simulink library "halout"  (R2021b)
settings: Solver=VariableStepAuto  StartTime=0.0  StopTime=10.0  RelTol=1e-3
undefined symbols (not defined in the file): C_TASK_5MS_S, FALSE, KHAL_CAN1FD1APS3E2E_flg, KHAL_CAN1FD1APS3TxReq_flg, KHAL_CAN1FD1VCU2E2E_flg, KHAL_CAN1FD1VCU2TxReq_flg, KHAL_CAN1FD1VCU3E2E_flg, KHAL_CAN1FD1VCU3TxReq_flg, KHAL_CAN1TxReq_flg, KHAL_CAN1VMCFCM1E2E_flg, KHAL_CAN1VMCFCM1TxReq_flg, KHAL_CAN2TxReq_flg, KHAL_CAN3FD3VCU1toNIDECTxReq_flg, KHAL_CAN3FD3VCU1TxReq_flg, KHAL_CAN3FD3VCU2E2E_flg, KHAL_CAN3FD3VCU2toNIDECE2E_flg, KHAL_CAN3FD3VCU2toNIDECTxReq_flg, KHAL_CAN3FD3VCU2TxReq_flg, KHAL_CAN3TxReq_flg, KHAL_CAN4FD4CE1000E2E_flg, KHAL_CAN4FD4CE1000TxReq_flg, KHAL_CAN4TxReq_flg, KHAL_CAN5TxReq_flg, KHAL_CAN6FD6APS3E2E_flg, KHAL_CAN6FD6APS3TxReq_flg, KHAL_CAN6FD6VCU2E2E_flg, KHAL_CAN6FD6VCU2TxReq_flg, KHAL_CAN6TxReq_flg, ONE_INT, TRUE, ZERO_INT
libraries: FVT_lib x551, simulink x244
(part 24 of 26)

== system halout/HAL_OUT/CAN5/FD5_Debug2_0x4F7/FDCDKCRemoRightPSDCmd ==
  FDCDKCRemoRightPSDCmd : Inport
  Data Type Conversion : DataTypeConversion  OutDataTypeStr=uint8  RndMeth=Round
  CAN5_FDC_DKC_RemoRightPSD_Cmd : Outport
  wires:
  Data Type Conversion/1 -> CAN5_FDC_DKC_RemoRightPSD_Cmd/1
  FDCDKCRemoRightPSDCmd/1 -> Data Type Conversion/1

== system halout/HAL_OUT/CAN5/FD5_Debug2_0x4F7/FDCDKCSPTGDetCmd ==
  FDCDKCSPTGDetCmd : Inport
  Data Type Conversion : DataTypeConversion  OutDataTypeStr=uint8  RndMeth=Round
  CAN5_FDC_DKC_SPTGDet_Cmd : Outport
  wires:
  Data Type Conversion/1 -> CAN5_FDC_DKC_SPTGDet_Cmd/1
  FDCDKCSPTGDetCmd/1 -> Data Type Conversion/1

== system halout/HAL_OUT/CAN5/FD5_Debug2_0x4F7/FDCDKCSPTGOpenCmd ==
  FDCDKCSPTGOpenCmd : Inport
  Data Type Conversion : DataTypeConversion  OutDataTypeStr=uint8  RndMeth=Round
  CAN5_FDC_DKC_SPTGOpen_Cmd : Outport
  wires:
  Data Type Conversion/1 -> CAN5_FDC_DKC_SPTGOpen_Cmd/1
  FDCDKCSPTGOpenCmd/1 -> Data Type Conversion/1

== system halout/HAL_OUT/CAN5/FD5_Debug2_0x4F7/FDCDKCShippingModeSta ==
  FDCDKCShippingModeSta : Inport
  Data Type Conversion : DataTypeConversion  OutDataTypeStr=uint8  RndMeth=Round
  CAN5_FDC_DKC_ShippingMode_Sta : Outport
  wires:
  Data Type Conversion/1 -> CAN5_FDC_DKC_ShippingMode_Sta/1
  FDCDKCShippingModeSta/1 -> Data Type Conversion/1

== system halout/HAL_OUT/CAN5/FD5_Debug2_0x4F7/FDCDKCUIDBatVoltSta ==
  FDCDKCUIDBatVoltSta : Inport
  Data Type Conversion : DataTypeConversion  OutDataTypeStr=uint16  RndMeth=Round
  convert_out : FVT_lib/hal/convert_out  gain=10  offset=0
  CAN5_FDC_DKC_UIDBatVolt_Sta : Outport
  wires:
  Data Type Conversion/1 -> CAN5_FDC_DKC_UIDBatVolt_Sta/1
  convert_out/1 -> Data Type Conversion/1
  FDCDKCUIDBatVoltSta/1 -> convert_out/1

== system halout/HAL_OUT/CAN5/FD5_Debug2_0x4F7/FDCDKCUIDLowPowerSta ==
  FDCDKCUIDLowPowerSta : Inport
  Data Type Conversion : DataTypeConversion  OutDataTypeStr=uint8  RndMeth=Round
  CAN5_FDC_DKC_UIDLowPower_Sta : Outport
  wires:
  Data Type Conversion/1 -> CAN5_FDC_DKC_UIDLowPower_Sta/1
  FDCDKCUIDLowPowerSta/1 -> Data Type Conversion/1

== system halout/HAL_OUT/CAN5/FD5_Debug2_0x4F7/FDCDKCUWB1DistanceSta ==
  FDCDKCUWB1DistanceSta : Inport
  Data Type Conversion : DataTypeConversion  OutDataTypeStr=uint8  RndMeth=Round
  convert_out : FVT_lib/hal/convert_out  gain=10  offset=0
  CAN5_FDC_DKC_UWB1_Distance_Sta : Outport
  wires:
  Data Type Conversion/1 -> CAN5_FDC_DKC_UWB1_Distance_Sta/1
  convert_out/1 -> Data Type Conversion/1
  FDCDKCUWB1DistanceSta/1 -> convert_out/1

== system halout/HAL_OUT/CAN5/FD5_Debug2_0x4F7/FDCDKCUWB1FPPSta ==
  FDCDKCUWB1FPPSta : Inport
  Data Type Conversion : DataTypeConversion  OutDataTypeStr=uint8  RndMeth=Round
  convert_out : FVT_lib/hal/convert_out  gain=1  offset=-127
  CAN5_FDC_DKC_UWB1_FPP_Sta : Outport
  wires:
  Data Type Conversion/1 -> CAN5_FDC_DKC_UWB1_FPP_Sta/1
  convert_out/1 -> Data Type Conversion/1
  FDCDKCUWB1FPPSta/1 -> convert_out/1

== system halout/HAL_OUT/CAN5/FD5_Debug2_0x4F7/FDCDKCUWB1InvalidSta ==
  FDCDKCUWB1InvalidSta : Inport
  Data Type Conversion : DataTypeConversion  OutDataTypeStr=uint8  RndMeth=Round
  CAN5_FDC_DKC_UWB1_Invalid_Sta : Outport
  wires:
  Data Type Conversion/1 -> CAN5_FDC_DKC_UWB1_Invalid_Sta/1
  FDCDKCUWB1InvalidSta/1 -> Data Type Conversion/1

== system halout/HAL_OUT/CAN5/FD5_Debug2_0x4F7/FDCDKCUWB2DistanceSta ==
  FDCDKCUWB2DistanceSta : Inport
  Data Type Conversion : DataTypeConversion  OutDataTypeStr=uint8  RndMeth=Round
  convert_out : FVT_lib/hal/convert_out  gain=10  offset=0
  CAN5_FDC_DKC_UWB2_Distance_Sta : Outport
  wires:
  Data Type Conversion/1 -> CAN5_FDC_DKC_UWB2_Distance_Sta/1
  convert_out/1 -> Data Type Conversion/1
  FDCDKCUWB2DistanceSta/1 -> convert_out/1

== system halout/HAL_OUT/CAN5/FD5_Debug2_0x4F7/FDCDKCUWB2FPPSta ==
  FDCDKCUWB2FPPSta : Inport
  Data Type Conversion : DataTypeConversion  OutDataTypeStr=uint8  RndMeth=Round
  convert_out : FVT_lib/hal/convert_out  gain=1  offset=-127
  CAN5_FDC_DKC_UWB2_FPP_Sta : Outport
  wires:
  Data Type Conversion/1 -> CAN5_FDC_DKC_UWB2_FPP_Sta/1
  convert_out/1 -> Data Type Conversion/1
  FDCDKCUWB2FPPSta/1 -> convert_out/1

== system halout/HAL_OUT/CAN5/FD5_Debug2_0x4F7/FDCDKCUWB2InvalidSta ==
  FDCDKCUWB2InvalidSta : Inport
  Data Type Conversion : DataTypeConversion  OutDataTypeStr=uint8  RndMeth=Round
  CAN5_FDC_DKC_UWB2_Invalid_Sta : Outport
  wires:
  Data Type Conversion/1 -> CAN5_FDC_DKC_UWB2_Invalid_Sta/1
  FDCDKCUWB2InvalidSta/1 -> Data Type Conversion/1

== system halout/HAL_OUT/CAN5/FD5_Debug2_0x4F7/FDCDKCUWB3DistanceSta ==
  FDCDKCUWB3DistanceSta : Inport
  Data Type Conversion : DataTypeConversion  OutDataTypeStr=uint8  RndMeth=Round
  convert_out : FVT_lib/hal/convert_out  gain=10  offset=0
  CAN5_FDC_DKC_UWB3_Distance_Sta : Outport
  wires:
  Data Type Conversion/1 -> CAN5_FDC_DKC_UWB3_Distance_Sta/1
  convert_out/1 -> Data Type Conversion/1
  FDCDKCUWB3DistanceSta/1 -> convert_out/1

== system halout/HAL_OUT/CAN5/FD5_Debug2_0x4F7/FDCDKCUWB3FPPSta ==
  FDCDKCUWB3FPPSta : Inport
  Data Type Conversion : DataTypeConversion  OutDataTypeStr=uint8  RndMeth=Round
  convert_out : FVT_lib/hal/convert_out  gain=1  offset=-127
  CAN5_FDC_DKC_UWB3_FPP_Sta : Outport
  wires:
  Data Type Conversion/1 -> CAN5_FDC_DKC_UWB3_FPP_Sta/1
  convert_out/1 -> Data Type Conversion/1
  FDCDKCUWB3FPPSta/1 -> convert_out/1

== system halout/HAL_OUT/CAN5/FD5_Debug2_0x4F7/FDCDKCUWB3InvalidSta ==
  FDCDKCUWB3InvalidSta : Inport
  Data Type Conversion : DataTypeConversion  OutDataTypeStr=uint8  RndMeth=Round
  CAN5_FDC_DKC_UWB3_Invalid_Sta : Outport
  wires:
  Data Type Conversion/1 -> CAN5_FDC_DKC_UWB3_Invalid_Sta/1
  FDCDKCUWB3InvalidSta/1 -> Data Type Conversion/1

== system halout/HAL_OUT/CAN5/FD5_Debug2_0x4F7/FDCDKCUWB4DistanceSta ==
  FDCDKCUWB4DistanceSta : Inport
  Data Type Conversion : DataTypeConversion  OutDataTypeStr=uint8  RndMeth=Round
  convert_out : FVT_lib/hal/convert_out  gain=10  offset=0
  CAN5_FDC_DKC_UWB4_Distance_Sta : Outport
  wires:
  Data Type Conversion/1 -> CAN5_FDC_DKC_UWB4_Distance_Sta/1
  convert_out/1 -> Data Type Conversion/1
  FDCDKCUWB4DistanceSta/1 -> convert_out/1

== system halout/HAL_OUT/CAN5/FD5_Debug2_0x4F7/FDCDKCUWB4FPPSta ==
  FDCDKCUWB4FPPSta : Inport
  Data Type Conversion : DataTypeConversion  OutDataTypeStr=uint8  RndMeth=Round
  convert_out : FVT_lib/hal/convert_out  gain=1  offset=-127
  CAN5_FDC_DKC_UWB4_FPP_Sta : Outport
  wires:
  Data Type Conversion/1 -> CAN5_FDC_DKC_UWB4_FPP_Sta/1
  convert_out/1 -> Data Type Conversion/1
  FDCDKCUWB4FPPSta/1 -> convert_out/1

== system halout/HAL_OUT/CAN5/FD5_Debug2_0x4F7/FDCDKCUWB4InvalidSta ==
  FDCDKCUWB4InvalidSta : Inport
  Data Type Conversion : DataTypeConversion  OutDataTypeStr=uint8  RndMeth=Round
  CAN5_FDC_DKC_UWB4_Invalid_Sta : Outport
  wires:
  Data Type Conversion/1 -> CAN5_FDC_DKC_UWB4_Invalid_Sta/1
  FDCDKCUWB4InvalidSta/1 -> Data Type Conversion/1

== system halout/HAL_OUT/CAN5/FD5_Debug2_0x4F7/FDCDKCUWB5DistanceSta ==
  FDCDKCUWB5DistanceSta : Inport
  Data Type Conversion : DataTypeConversion  OutDataTypeStr=uint8  RndMeth=Round
  convert_out : FVT_lib/hal/convert_out  gain=10  offset=0
  CAN5_FDC_DKC_UWB5_Distance_Sta : Outport
  wires:
  Data Type Conversion/1 -> CAN5_FDC_DKC_UWB5_Distance_Sta/1
  convert_out/1 -> Data Type Conversion/1
  FDCDKCUWB5DistanceSta/1 -> convert_out/1

== system halout/HAL_OUT/CAN5/FD5_Debug2_0x4F7/FDCDKCUWB5FPPSta ==
  FDCDKCUWB5FPPSta : Inport
  Data Type Conversion : DataTypeConversion  OutDataTypeStr=uint8  RndMeth=Round
  convert_out : FVT_lib/hal/convert_out  gain=1  offset=-127
  CAN5_FDC_DKC_UWB5_FPP_Sta : Outport
  wires:
  Data Type Conversion/1 -> CAN5_FDC_DKC_UWB5_FPP_Sta/1
  convert_out/1 -> Data Type Conversion/1
  FDCDKCUWB5FPPSta/1 -> convert_out/1

== system halout/HAL_OUT/CAN5/FD5_Debug2_0x4F7/FDCDKCUWB5InvalidSta ==
  FDCDKCUWB5InvalidSta : Inport
  Data Type Conversion : DataTypeConversion  OutDataTypeStr=uint8  RndMeth=Round
  CAN5_FDC_DKC_UWB5_Invalid_Sta : Outport
  wires:
  Data Type Conversion/1 -> CAN5_FDC_DKC_UWB5_Invalid_Sta/1
  FDCDKCUWB5InvalidSta/1 -> Data Type Conversion/1

== system halout/HAL_OUT/CAN5/FD5_Debug2_0x4F7/FDCDKCUWBDetAreaSta ==
  FDCDKCUWBDetAreaSta : Inport
  Data Type Conversion : DataTypeConversion  OutDataTypeStr=uint8  RndMeth=Round
  CAN5_FDC_DKC_UWBDetArea_Sta : Outport
  wires:
  Data Type Conversion/1 -> CAN5_FDC_DKC_UWBDetArea_Sta/1
  FDCDKCUWBDetAreaSta/1 -> Data Type Conversion/1

== system halout/HAL_OUT/CAN5/FD5_Debug2_0x4F7/FDCDKCUWBDetPTGAreaSta ==
  FDCDKCUWBDetPTGAreaSta : Inport
  Data Type Conversion : DataTypeConversion  OutDataTypeStr=uint8  RndMeth=Round
  CAN5_FDC_DKC_UWBDetPTGArea_Sta : Outport
  wires:
  Data Type Conversion/1 -> CAN5_FDC_DKC_UWBDetPTGArea_Sta/1
  FDCDKCUWBDetPTGAreaSta/1 -> Data Type Conversion/1

== system halout/HAL_OUT/CAN5/FD5_Debug2_0x4F7/FDCDKCUWBOnOffSta ==
  FDCDKCUWBOnOffSta : Inport
  Data Type Conversion : DataTypeConversion  OutDataTypeStr=uint8  RndMeth=Round
  CAN5_FDC_DKC_UWB_OnOff_Sta : Outport
  wires:
  Data Type Conversion/1 -> CAN5_FDC_DKC_UWB_OnOff_Sta/1
  FDCDKCUWBOnOffSta/1 -> Data Type Conversion/1

== system halout/HAL_OUT/CAN5/FD5_Debug3_0x4F3/FDCVMCActReqAccCmd ==
  FDCVMCActReqAccCmd : Inport
  Data Type Conversion : DataTypeConversion  OutDataTypeStr=uint16  RndMeth=Round
  convert_out : FVT_lib/hal/convert_out  gain=0.05  offset=-15
  CAN5_FDC_VMC_ActReqAcc_Cmd : Outport
  wires:
  Data Type Conversion/1 -> CAN5_FDC_VMC_ActReqAcc_Cmd/1
  convert_out/1 -> Data Type Conversion/1
  FDCVMCActReqAccCmd/1 -> convert_out/1

== system halout/HAL_OUT/CAN5/FD5_Debug3_0x4F3/FDCVMCExtraMSACtrlSta ==
  FDCVMCExtraMSACtrlSta : Inport
  Data Type Conversion : DataTypeConversion  OutDataTypeStr=uint8  RndMeth=Round
  CAN5_FDC_VMC_ExtraMSACtrl_Sta : Outport
  wires:
  Data Type Conversion/1 -> CAN5_FDC_VMC_ExtraMSACtrl_Sta/1
  FDCVMCExtraMSACtrlSta/1 -> Data Type Conversion/1

== system halout/HAL_OUT/CAN5/FD5_Debug3_0x4F3/FDCVMCIMUGxCmd ==
  FDCVMCIMUGxCmd : Inport
  Data Type Conversion : DataTypeConversion  OutDataTypeStr=uint8  RndMeth=Round
  convert_out : FVT_lib/hal/convert_out  gain=0.01  offset=-1.27
  CAN5_FDC_VMC_IMUGx_Cmd : Outport
  wires:
  Data Type Conversion/1 -> CAN5_FDC_VMC_IMUGx_Cmd/1
  convert_out/1 -> Data Type Conversion/1
  FDCVMCIMUGxCmd/1 -> convert_out/1

== system halout/HAL_OUT/CAN5/FD5_Debug3_0x4F3/FDCVMCIMUGyCmd ==
  FDCVMCIMUGyCmd : Inport
  Data Type Conversion : DataTypeConversion  OutDataTypeStr=uint8  RndMeth=Round
  convert_out : FVT_lib/hal/convert_out  gain=0.01  offset=-1.27
  CAN5_FDC_VMC_IMUGy_Cmd : Outport
  wires:
  Data Type Conversion/1 -> CAN5_FDC_VMC_IMUGy_Cmd/1
  convert_out/1 -> Data Type Conversion/1
  FDCVMCIMUGyCmd/1 -> convert_out/1

== system halout/HAL_OUT/CAN5/FD5_Debug3_0x4F3/FDCVMCIMUGzCmd ==
  FDCVMCIMUGzCmd : Inport
  Data Type Conversion : DataTypeConversion  OutDataTypeStr=uint8  RndMeth=Round
  convert_out : FVT_lib/hal/convert_out  gain=0.01  offset=-1.27
  CAN5_FDC_VMC_IMUGz_Cmd : Outport
  wires:
  Data Type Conversion/1 -> CAN5_FDC_VMC_IMUGz_Cmd/1
  convert_out/1 -> Data Type Conversion/1
  FDCVMCIMUGzCmd/1 -> convert_out/1

== system halout/HAL_OUT/CAN5/FD5_Debug3_0x4F3/FDCVMCIMUPitchRateCmd ==
  FDCVMCIMUPitchRateCmd : Inport
  Data Type Conversion : DataTypeConversion  OutDataTypeStr=uint16  RndMeth=Round
  convert_out : FVT_lib/hal/convert_out  gain=0.1  offset=-100
  CAN5_FDC_VMC_IMUPitchRate_Cmd : Outport
  wires:
  Data Type Conversion/1 -> CAN5_FDC_VMC_IMUPitchRate_Cmd/1
  convert_out/1 -> Data Type Conversion/1
  FDCVMCIMUPitchRateCmd/1 -> convert_out/1

== system halout/HAL_OUT/CAN5/FD5_Debug3_0x4F3/FDCVMCIMURollRateCmd ==
  FDCVMCIMURollRateCmd : Inport
  Data Type Conversion : DataTypeConversion  OutDataTypeStr=uint16  RndMeth=Round
  convert_out : FVT_lib/hal/convert_out  gain=0.1  offset=-100
  CAN5_FDC_VMC_IMURollRate_Cmd : Outport
  wires:
  Data Type Conversion/1 -> CAN5_FDC_VMC_IMURollRate_Cmd/1
  convert_out/1 -> Data Type Conversion/1
  FDCVMCIMURollRateCmd/1 -> convert_out/1

== system halout/HAL_OUT/CAN5/FD5_Debug3_0x4F3/FDCVMCIMUYawRateCmd ==
  FDCVMCIMUYawRateCmd : Inport
  Data Type Conversion : DataTypeConversion  OutDataTypeStr=uint16  RndMeth=Round
  convert_out : FVT_lib/hal/convert_out  gain=0.1  offset=-100
  CAN5_FDC_VMC_IMUYawRate_Cmd : Outport
  wires:
  Data Type Conversion/1 -> CAN5_FDC_VMC_IMUYawRate_Cmd/1
  convert_out/1 -> Data Type Conversion/1
  FDCVMCIMUYawRateCmd/1 -> convert_out/1

== system halout/HAL_OUT/CAN5/FD5_Debug3_0x4F3/FDCVMCLongAccelCmd ==
  FDCVMCLongAccelCmd : Inport
  Data Type Conversion : DataTypeConversion  OutDataTypeStr=uint8  RndMeth=Round
  convert_out : FVT_lib/hal/convert_out  gain=0.01  offset=-1.27
  CAN5_FDC_VMC_LongAccel_Cmd : Outport
  wires:
  Data Type Conversion/1 -> CAN5_FDC_VMC_LongAccel_Cmd/1
  convert_out/1 -> Data Type Conversion/1
  FDCVMCLongAccelCmd/1 -> convert_out/1

== system halout/HAL_OUT/CAN5/GW5_CE100_0_0x1C5/FDCBCMWinLFOpenedSta ==
  FDCBCMWinLFOpenedSta : Inport
  Data Type Conversion : DataTypeConversion  OutDataTypeStr=uint8  RndMeth=Round
  CAN5_FDC_BCM_WinLFOpened_Sta : Outport
  wires:
  Data Type Conversion/1 -> CAN5_FDC_BCM_WinLFOpened_Sta/1
  FDCBCMWinLFOpenedSta/1 -> Data Type Conversion/1

== system halout/HAL_OUT/CAN5/GW5_CE100_0_0x1C5/FDCBCMWinLROpenedSta ==
  FDCBCMWinLROpenedSta : Inport
  Data Type Conversion : DataTypeConversion  OutDataTypeStr=uint8  RndMeth=Round
  CAN5_FDC_BCM_WinLROpened_Sta : Outport
  wires:
  Data Type Conversion/1 -> CAN5_FDC_BCM_WinLROpened_Sta/1
  FDCBCMWinLROpenedSta/1 -> Data Type Conversion/1

== system halout/HAL_OUT/CAN5/GW5_CE100_0_0x1C5/FDCBCMWinRFOpenedSta ==
  FDCBCMWinRFOpenedSta : Inport
  Data Type Conversion : DataTypeConversion  OutDataTypeStr=uint8  RndMeth=Round
  CAN5_FDC_BCM_WinRFOpened_Sta : Outport
  wires:
  Data Type Conversion/1 -> CAN5_FDC_BCM_WinRFOpened_Sta/1
  FDCBCMWinRFOpenedSta/1 -> Data Type Conversion/1

== system halout/HAL_OUT/CAN5/GW5_CE100_0_0x1C5/FDCBCMWinRROpenedSta ==
  FDCBCMWinRROpenedSta : Inport
  Data Type Conversion : DataTypeConversion  OutDataTypeStr=uint8  RndMeth=Round
  CAN5_FDC_BCM_WinRROpened_Sta : Outport
  wires:
  Data Type Conversion/1 -> CAN5_FDC_BCM_WinRROpened_Sta/1
  FDCBCMWinRROpenedSta/1 -> Data Type Conversion/1

== system halout/HAL_OUT/CAN6/FD6_APS3_0x238/APS3LifeCount ==
  APS3LifeCount : Inport
  Data Type Conversion : DataTypeConversion  OutDataTypeStr=uint8  RndMeth=Round
  CAN6_APS3_LifeCount : Outport
  wires:
  Data Type Conversion/1 -> CAN6_APS3_LifeCount/1
  APS3LifeCount/1 -> Data Type Conversion/1

== system halout/HAL_OUT/CAN6/FD6_APS3_0x238/APS3checksum ==
  APS3checksum : Inport
  Data Type Conversion : DataTypeConversion  OutDataTypeStr=uint8  RndMeth=Round
  CAN6_APS3_checksum : Outport
  wires:
  Data Type Conversion/1 -> CAN6_APS3_checksum/1
  APS3checksum/1 -> Data Type Conversion/1

== system halout/HAL_OUT/CAN6/FD6_APS3_0x238/APSDecReq ==
  APSDecReq : Inport
  Data Type Conversion : DataTypeConversion  OutDataTypeStr=uint8  RndMeth=Round
  convert_out : FVT_lib/hal/convert_out  gain=0.1  offset=0
  CAN6_APS_DecReq : Outport
  wires:
  Data Type Conversion/1 -> CAN6_APS_DecReq/1
  convert_out/1 -> Data Type Conversion/1
  APSDecReq/1 -> convert_out/1

== system halout/HAL_OUT/CAN6/FD6_APS3_0x238/APSDecReqA ==
  APSDecReqA : Inport
  Data Type Conversion : DataTypeConversion  OutDataTypeStr=uint8  RndMeth=Round
  CAN6_APS_DecReq_A : Outport
  wires:
  Data Type Conversion/1 -> CAN6_APS_DecReq_A/1
  APSDecReqA/1 -> Data Type Conversion/1

== system halout/HAL_OUT/CAN6/FD6_APS3_0x238/APSOpenPTG ==
  APSOpenPTG : Inport
  Data Type Conversion : DataTypeConversion  OutDataTypeStr=uint8  RndMeth=Round
  CAN6_APSOpenPTG : Outport
  wires:
  Data Type Conversion/1 -> CAN6_APSOpenPTG/1
  APSOpenPTG/1 -> Data Type Conversion/1

== system halout/HAL_OUT/CAN6/FD6_APS3_0x238/APSReq ==
  APSReq : Inport
  Data Type Conversion : DataTypeConversion  OutDataTypeStr=uint8  RndMeth=Round
  CAN6_APS_Req : Outport
  wires:
  Data Type Conversion/1 -> CAN6_APS_Req/1
  APSReq/1 -> Data Type Conversion/1

== system halout/HAL_OUT/CAN6/FD6_APS3_0x238/APSStaSystem ==
  APSStaSystem : Inport
  Data Type Conversion : DataTypeConversion  OutDataTypeStr=uint8  RndMeth=Round
  CAN6_APS_Sta_System : Outport
  wires:
  Data Type Conversion/1 -> CAN6_APS_Sta_System/1
  APSStaSystem/1 -> Data Type Conversion/1

== system halout/HAL_OUT/CAN6/FD6_APS3_0x238/Byte_0 ==
  APS3_checksum : Inport
  BitwiseOR : simulink/Logic and Bit Operations/Bitwise Operator  logicop=OR  UseBitMask=off  BitMask=bin2dec('11011001')  BitMaskRealWorld=Stored Integer
  SignalPack : FVT_lib/hal/SignalPack  RightShiftCnt=0  BitMask=2^8-1  LeftShiftCnt=0
  UnitConverter : DataTypeConversion  OutDataTypeStr=uint8  RndMeth=Round
  UnitConverter1 : DataTypeConversion  OutDataTypeStr=uint8  RndMeth=Round
  Byte_0 : Outport
  wires:
  BitwiseOR/1 -> Byte_0/1
  UnitConverter/1 -> BitwiseOR/1
  SignalPack/1 -> UnitConverter/1
  UnitConverter1/1 -> SignalPack/1
  APS3_checksum/1 -> UnitConverter1/1

== system halout/HAL_OUT/CAN6/FD6_APS3_0x238/Byte_1 ==
  APS3_LifeCount : Inport
  BitwiseOR : simulink/Logic and Bit Operations/Bitwise Operator  logicop=OR  UseBitMask=off  BitMask=bin2dec('11011001')  BitMaskRealWorld=Stored Integer
  SignalPack : FVT_lib/hal/SignalPack  RightShiftCnt=0  BitMask=2^4-1  LeftShiftCnt=0
  UnitConverter : DataTypeConversion  OutDataTypeStr=uint8  RndMeth=Round
  UnitConverter1 : DataTypeConversion  OutDataTypeStr=uint8  RndMeth=Round
  Byte_1 : Outport
  wires:
  BitwiseOR/1 -> Byte_1/1
  UnitConverter/1 -> BitwiseOR/1
  SignalPack/1 -> UnitConverter/1
  UnitConverter1/1 -> SignalPack/1
  APS3_LifeCount/1 -> UnitConverter1/1

== system halout/HAL_OUT/CAN6/FD6_APS3_0x238/Byte_2 ==
  APSOpenPTG : Inport
  APS_DecReq_A : Inport  Port=2
  APS_Req : Inport  Port=3
  CAAS_Sta : Inport  Port=4
  BitwiseOR : simulink/Logic and Bit Operations/Bitwise Operator  logicop=OR  UseBitMask=off  NumInputPorts=4  BitMask=bin2dec('11011001')  BitMaskRealWorld=Stored Integer
  SignalPack : FVT_lib/hal/SignalPack  RightShiftCnt=0  BitMask=2^1-1  LeftShiftCnt=0
  SignalPack1 : FVT_lib/hal/SignalPack  RightShiftCnt=0  BitMask=2^1-1  LeftShiftCnt=7
  SignalPack2 : FVT_lib/hal/SignalPack  RightShiftCnt=0  BitMask=2^3-1  LeftShiftCnt=4
  SignalPack3 : FVT_lib/hal/SignalPack  RightShiftCnt=0  BitMask=2^3-1  LeftShiftCnt=1
  UnitConverter{,1..7} (8 alike) : DataTypeConversion  OutDataTypeStr=uint8  RndMeth=Round
  Byte_2 : Outport
  wires:
  BitwiseOR/1 -> Byte_2/1
  UnitConverter/1 -> BitwiseOR/1
  SignalPack/1 -> UnitConverter/1
  UnitConverter1/1 -> SignalPack/1
  APSOpenPTG/1 -> UnitConverter1/1
  UnitConverter2/1 -> BitwiseOR/2
  SignalPack1/1 -> UnitConverter2/1
  UnitConverter3/1 -> SignalPack1/1
  APS_DecReq_A/1 -> UnitConverter3/1
  UnitConverter4/1 -> BitwiseOR/3
  SignalPack2/1 -> UnitConverter4/1
  UnitConverter5/1 -> SignalPack2/1
  APS_Req/1 -> UnitConverter5/1
  UnitConverter6/1 -> BitwiseOR/4
  SignalPack3/1 -> UnitConverter6/1
  UnitConverter7/1 -> SignalPack3/1
  CAAS_Sta/1 -> UnitConverter7/1

== system halout/HAL_OUT/CAN6/FD6_APS3_0x238/Byte_3 ==
  APS_DecReq : Inport
  BitwiseOR : simulink/Logic and Bit Operations/Bitwise Operator  logicop=OR  UseBitMask=off  BitMask=bin2dec('11011001')  BitMaskRealWorld=Stored Integer
  SignalPack : FVT_lib/hal/SignalPack  RightShiftCnt=0  BitMask=2^8-1  LeftShiftCnt=0
  UnitConverter : DataTypeConversion  OutDataTypeStr=uint8  RndMeth=Round
  UnitConverter1 : DataTypeConversion  OutDataTypeStr=uint8  RndMeth=Round
  convert_out : FVT_lib/hal/convert_out  gain=0.1  offset=0
  Byte_3 : Outport
  wires:
  BitwiseOR/1 -> Byte_3/1
  UnitConverter/1 -> BitwiseOR/1
  SignalPack/1 -> UnitConverter/1
  UnitConverter1/1 -> SignalPack/1
  convert_out/1 -> UnitConverter1/1
  APS_DecReq/1 -> convert_out/1

== system halout/HAL_OUT/CAN6/FD6_APS3_0x238/Byte_4 ==
  FDC_VMC_APS_Angle_Target : Inport
  BitwiseOR : simulink/Logic and Bit Operations/Bitwise Operator  logicop=OR  UseBitMask=off  BitMask=bin2dec('11011001')  BitMaskRealWorld=Stored Integer
  SignalPack : FVT_lib/hal/SignalPack  RightShiftCnt=8  BitMask=2^8-1  LeftShiftCnt=0
  UnitConverter : DataTypeConversion  OutDataTypeStr=uint8  RndMeth=Round
  UnitConverter1 : DataTypeConversion  OutDataTypeStr=uint16  RndMeth=Round
  convert_out : FVT_lib/hal/convert_out  gain=0.1  offset=-900
  Byte_4 : Outport
  wires:
  BitwiseOR/1 -> Byte_4/1
  UnitConverter/1 -> BitwiseOR/1
  SignalPack/1 -> UnitConverter/1
  UnitConverter1/1 -> SignalPack/1
  convert_out/1 -> UnitConverter1/1
  FDC_VMC_APS_Angle_Target/1 -> convert_out/1

== system halout/HAL_OUT/CAN6/FD6_APS3_0x238/Byte_5 ==
  FDC_VMC_APS_Angle_Target : Inport
  BitwiseOR : simulink/Logic and Bit Operations/Bitwise Operator  logicop=OR  UseBitMask=off  BitMask=bin2dec('11011001')  BitMaskRealWorld=Stored Integer
  SignalPack : FVT_lib/hal/SignalPack  RightShiftCnt=0  BitMask=2^8-1  LeftShiftCnt=0
  UnitConverter : DataTypeConversion  OutDataTypeStr=uint8  RndMeth=Round
  UnitConverter1 : DataTypeConversion  OutDataTypeStr=uint16  RndMeth=Round
  convert_out : FVT_lib/hal/convert_out  gain=0.1  offset=-900
  Byte_5 : Outport
  wires:
  BitwiseOR/1 -> Byte_5/1
  UnitConverter/1 -> BitwiseOR/1
  SignalPack/1 -> UnitConverter/1
  UnitConverter1/1 -> SignalPack/1
  convert_out/1 -> UnitConverter1/1
  FDC_VMC_APS_Angle_Target/1 -> convert_out/1

== system halout/HAL_OUT/CAN6/FD6_APS3_0x238/Byte_6 ==
  APS_Sta_System : Inport
  FDC_VMC_APS_V_Rq_EPS_Ctrl : Inport  Port=2
  SPTGDet : Inport  Port=3
  SPTG_Sta : Inport  Port=4
  BitwiseOR : simulink/Logic and Bit Operations/Bitwise Operator  logicop=OR  UseBitMask=off  NumInputPorts=4  BitMask=bin2dec('11011001')  BitMaskRealWorld=Stored Integer
  SignalPack : FVT_lib/hal/SignalPack  RightShiftCnt=0  BitMask=2^3-1  LeftShiftCnt=0
  SignalPack1 : FVT_lib/hal/SignalPack  RightShiftCnt=0  BitMask=2^1-1  LeftShiftCnt=3
  SignalPack2 : FVT_lib/hal/SignalPack  RightShiftCnt=0  BitMask=2^1-1  LeftShiftCnt=7
  SignalPack3 : FVT_lib/hal/SignalPack  RightShiftCnt=0  BitMask=2^3-1  LeftShiftCnt=4
  UnitConverter{,1..7} (8 alike) : DataTypeConversion  OutDataTypeStr=uint8  RndMeth=Round
  Byte_6 : Outport
  wires:
  BitwiseOR/1 -> Byte_6/1
  UnitConverter/1 -> BitwiseOR/1
  SignalPack/1 -> UnitConverter/1
  UnitConverter1/1 -> SignalPack/1
  APS_Sta_System/1 -> UnitConverter1/1
  UnitConverter2/1 -> BitwiseOR/2
  SignalPack1/1 -> UnitConverter2/1
  UnitConverter3/1 -> SignalPack1/1
  FDC_VMC_APS_V_Rq_EPS_Ctrl/1 -> UnitConverter3/1
  UnitConverter4/1 -> BitwiseOR/3
  SignalPack2/1 -> UnitConverter4/1
  UnitConverter5/1 -> SignalPack2/1
  SPTGDet/1 -> UnitConverter5/1
  UnitConverter6/1 -> BitwiseOR/4
  SignalPack3/1 -> UnitConverter6/1
  UnitConverter7/1 -> SignalPack3/1
  SPTG_Sta/1 -> UnitConverter7/1

== system halout/HAL_OUT/CAN6/FD6_APS3_0x238/Byte_7 ==
  FDC_VMC_APS_Rq_EPS_Ctrl : Inport
  BitwiseOR : simulink/Logic and Bit Operations/Bitwise Operator  logicop=OR  UseBitMask=off  BitMask=bin2dec('11011001')  BitMaskRealWorld=Stored Integer
  SignalPack : FVT_lib/hal/SignalPack  RightShiftCnt=0  BitMask=2^1-1  LeftShiftCnt=0
  UnitConverter : DataTypeConversion  OutDataTypeStr=uint8  RndMeth=Round
  UnitConverter1 : DataTypeConversion  OutDataTypeStr=uint8  RndMeth=Round
  Byte_7 : Outport
  wires:
  BitwiseOR/1 -> Byte_7/1
  UnitConverter/1 -> BitwiseOR/1
  SignalPack/1 -> UnitConverter/1
  UnitConverter1/1 -> SignalPack/1
  FDC_VMC_APS_Rq_EPS_Ctrl/1 -> UnitConverter1/1

== system halout/HAL_OUT/CAN6/FD6_APS3_0x238/CAASSta ==
  CAASSta : Inport
  Data Type Conversion : DataTypeConversion  OutDataTypeStr=uint8  RndMeth=Round
  CAN6_CAAS_Sta : Outport
  wires:
  Data Type Conversion/1 -> CAN6_CAAS_Sta/1
  CAASSta/1 -> Data Type Conversion/1

== system halout/HAL_OUT/CAN6/FD6_APS3_0x238/CRC8_IfAction_Tx ==
  CAN_E2E_flg : Inport
  DataID1 : Inport  Port=2
  DataID2 : Inport  Port=3
  RawData : Inport  Port=4
  Data Type Conversion : DataTypeConversion  OutDataTypeStr=uint8
  If : If
  If Action Subsystem : Subsystem  TreatAsAtomicUnit=on
  If Action Subsystem1 : Subsystem  TreatAsAtomicUnit=on
  Merge : Merge
  CRC8 : Outport
  wires:
  If/2 -> If Action Subsystem/Action
  If/1 -> If Action Subsystem1/Action
  CAN_E2E_flg/1 -> [CAN_E2E_flg]
  DataID1/1 -> [DataID1]
  DataID2/1 -> [DataID2]
  RawData/1 -> [RawData]
  [CAN_E2E_flg] -> Data Type Conversion/1
  [DataID1] -> If Action Subsystem1/1(CAN_E2E_ID1)
  [DataID2] -> If Action Subsystem1/2(CAN_E2E_ID2)
  [RawData] -> If Action Subsystem1/3(Byte1)
  [RawData] -> If Action Subsystem/1(Byte1)
  If Action Subsystem1/1(CRC8_E2EResult) -> Merge/1
  If Action Subsystem/1(CRC8_Result) -> Merge/2
  Merge/1 -> CRC8/1
  Data Type Conversion/1 -> If/1

== system halout/HAL_OUT/CAN6/FD6_APS3_0x238/FDCVMCAPSAngleTarget ==
  FDCVMCAPSAngleTarget : Inport
  Data Type Conversion : DataTypeConversion  OutDataTypeStr=uint16  RndMeth=Round
  convert_out : FVT_lib/hal/convert_out  gain=0.1  offset=-900
  CAN6_FDC_VMC_APS_Angle_Target : Outport
  wires:
  Data Type Conversion/1 -> CAN6_FDC_VMC_APS_Angle_Target/1
  convert_out/1 -> Data Type Conversion/1
  FDCVMCAPSAngleTarget/1 -> convert_out/1

== system halout/HAL_OUT/CAN6/FD6_APS3_0x238/FDCVMCAPSRqEPSCtrl ==
  FDCVMCAPSRqEPSCtrl : Inport
  Data Type Conversion : DataTypeConversion  OutDataTypeStr=uint8  RndMeth=Round
  CAN6_FDC_VMC_APS_Rq_EPS_Ctrl : Outport
  wires:
  Data Type Conversion/1 -> CAN6_FDC_VMC_APS_Rq_EPS_Ctrl/1
  FDCVMCAPSRqEPSCtrl/1 -> Data Type Conversion/1

== system halout/HAL_OUT/CAN6/FD6_APS3_0x238/FDCVMCAPSVRqEPSCtrl ==
  FDCVMCAPSVRqEPSCtrl : Inport
  Data Type Conversion : DataTypeConversion  OutDataTypeStr=uint8  RndMeth=Round
  CAN6_FDC_VMC_APS_V_Rq_EPS_Ctrl : Outport
  wires:
  Data Type Conversion/1 -> CAN6_FDC_VMC_APS_V_Rq_EPS_Ctrl/1
  FDCVMCAPSVRqEPSCtrl/1 -> Data Type Conversion/1

== system halout/HAL_OUT/CAN6/FD6_APS3_0x238/SPTGDet ==
  SPTGDet : Inport
  Data Type Conversion : DataTypeConversion  OutDataTypeStr=uint8  RndMeth=Round
  CAN6_SPTGDet : Outport
  wires:
  Data Type Conversion/1 -> CAN6_SPTGDet/1
  SPTGDet/1 -> Data Type Conversion/1

== system halout/HAL_OUT/CAN6/FD6_APS3_0x238/SPTGSta ==
  SPTGSta : Inport
  Data Type Conversion : DataTypeConversion  OutDataTypeStr=uint8  RndMeth=Round
  CAN6_SPTG_Sta : Outport
  wires:
  Data Type Conversion/1 -> CAN6_SPTG_Sta/1
  SPTGSta/1 -> Data Type Conversion/1

== system halout/HAL_OUT/CAN6/FD6_BCM1_0x216/AllDoorSW ==
  AllDoorSW : Inport
  Data Type Conversion : DataTypeConversion  OutDataTypeStr=uint8  RndMeth=Round
  CAN6_AllDoorSW : Outport
  wires:
  Data Type Conversion/1 -> CAN6_AllDoorSW/1
  AllDoorSW/1 -> Data Type Conversion/1

== system halout/HAL_OUT/CAN6/FD6_BCM1_0x216/AntiTheftSeatFold ==
  AntiTheftSeatFold : Inport
  Data Type Conversion : DataTypeConversion  OutDataTypeStr=uint8  RndMeth=Round
  CAN6_AntiTheftSeatFold : Outport
  wires:
  Data Type Conversion/1 -> CAN6_AntiTheftSeatFold/1
  AntiTheftSeatFold/1 -> Data Type Conversion/1

== system halout/HAL_OUT/CAN6/FD6_BCM1_0x216/AntitheftSta ==
  AntitheftSta : Inport
  Data Type Conversion : DataTypeConversion  OutDataTypeStr=uint8  RndMeth=Round
  CAN6_AntitheftSta : Outport
  wires:
  Data Type Conversion/1 -> CAN6_AntitheftSta/1
  AntitheftSta/1 -> Data Type Conversion/1

== system halout/HAL_OUT/CAN6/FD6_BCM1_0x216/BCMBuzzerReq ==
  BCMBuzzerReq : Inport
  Data Type Conversion : DataTypeConversion  OutDataTypeStr=uint8  RndMeth=Round
  CAN6_BCM_Buzzer_Req : Outport
  wires:
  Data Type Conversion/1 -> CAN6_BCM_Buzzer_Req/1
  BCMBuzzerReq/1 -> Data Type Conversion/1

== system halout/HAL_OUT/CAN6/FD6_BCM1_0x216/BCMDoorLockSta ==
  BCMDoorLockSta : Inport
  Data Type Conversion : DataTypeConversion  OutDataTypeStr=uint8  RndMeth=Round
  CAN6_BCM_DoorLock_Sta : Outport
  wires:
  Data Type Conversion/1 -> CAN6_BCM_DoorLock_Sta/1
  BCMDoorLockSta/1 -> Data Type Conversion/1

== system halout/HAL_OUT/CAN6/FD6_BCM1_0x216/BrakeLamp ==
  BrakeLamp : Inport
  Data Type Conversion : DataTypeConversion  OutDataTypeStr=uint8  RndMeth=Round
  CAN6_BrakeLamp : Outport
  wires:
  Data Type Conversion/1 -> CAN6_BrakeLamp/1
  BrakeLamp/1 -> Data Type Conversion/1

== system halout/HAL_OUT/CAN6/FD6_BCM1_0x216/CTDCtrl ==
  CTDCtrl : Inport
  Data Type Conversion : DataTypeConversion  OutDataTypeStr=uint8  RndMeth=Round
  CAN6_CTDCtrl : Outport
  wires:
  Data Type Conversion/1 -> CAN6_CTDCtrl/1
  CTDCtrl/1 -> Data Type Conversion/1

== system halout/HAL_OUT/CAN6/FD6_BCM1_0x216/CTDLockSW ==
  CTDLockSW : Inport
  Data Type Conversion : DataTypeConversion  OutDataTypeStr=uint8  RndMeth=Round
  CAN6_CTDLockSW : Outport
  wires:
  Data Type Conversion/1 -> CAN6_CTDLockSW/1
  CTDLockSW/1 -> Data Type Conversion/1

== system halout/HAL_OUT/CAN6/FD6_BCM1_0x216/CTDUnlockSW ==
  CTDUnlockSW : Inport
  Data Type Conversion : DataTypeConversion  OutDataTypeStr=uint8  RndMeth=Round
  CAN6_CTDUnlockSW : Outport
  wires:
  Data Type Conversion/1 -> CAN6_CTDUnlockSW/1
  CTDUnlockSW/1 -> Data Type Conversion/1

== system halout/HAL_OUT/CAN6/FD6_BCM1_0x216/CrashDetd ==
  CrashDetd : Inport
  Data Type Conversion : DataTypeConversion  OutDataTypeStr=uint8  RndMeth=Round
  CAN6_CrashDetd : Outport
  wires:
  Data Type Conversion/1 -> CAN6_CrashDetd/1
  CrashDetd/1 -> Data Type Conversion/1

== system halout/HAL_OUT/CAN6/FD6_BCM1_0x216/Dimmer ==
  Dimmer : Inport
  Data Type Conversion : DataTypeConversion  OutDataTypeStr=uint8  RndMeth=Round
  CAN6_Dimmer : Outport
  wires:
  Data Type Conversion/1 -> CAN6_Dimmer/1
  Dimmer/1 -> Data Type Conversion/1

== system halout/HAL_OUT/CAN6/FD6_BCM1_0x216/DimmerEN ==
  DimmerEN : Inport
  Data Type Conversion : DataTypeConversion  OutDataTypeStr=uint8  RndMeth=Round
  CAN6_DimmerEN : Outport
  wires:
  Data Type Conversion/1 -> CAN6_DimmerEN/1
  DimmerEN/1 -> Data Type Conversion/1

== system halout/HAL_OUT/CAN6/FD6_BCM1_0x216/DoorLockIND ==
  DoorLockIND : Inport
  Data Type Conversion : DataTypeConversion  OutDataTypeStr=uint8  RndMeth=Round
  CAN6_DoorLockIND : Outport
  wires:
  Data Type Conversion/1 -> CAN6_DoorLockIND/1
  DoorLockIND/1 -> Data Type Conversion/1

== system halout/HAL_OUT/CAN6/FD6_BCM1_0x216/DrDoorSW ==
  DrDoorSW : Inport
  Data Type Conversion : DataTypeConversion  OutDataTypeStr=uint8  RndMeth=Round
  CAN6_DrDoorSW : Outport
  wires:
  Data Type Conversion/1 -> CAN6_DrDoorSW/1
  DrDoorSW/1 -> Data Type Conversion/1

== system halout/HAL_OUT/CAN6/FD6_BCM1_0x216/FrChargingDoorCtrl ==
  FrChargingDoorCtrl : Inport
  Data Type Conversion : DataTypeConversion  OutDataTypeStr=uint8  RndMeth=Round
  CAN6_Fr_ChargingDoorCtrl : Outport
  wires:
  Data Type Conversion/1 -> CAN6_Fr_ChargingDoorCtrl/1
  FrChargingDoorCtrl/1 -> Data Type Conversion/1

== system halout/HAL_OUT/CAN6/FD6_BCM1_0x216/FrFogLamp ==
  FrFogLamp : Inport
  Data Type Conversion : DataTypeConversion  OutDataTypeStr=uint8  RndMeth=Round
  CAN6_Fr_FogLamp : Outport
  wires:
  Data Type Conversion/1 -> CAN6_Fr_FogLamp/1
  FrFogLamp/1 -> Data Type Conversion/1

== system halout/HAL_OUT/CAN6/FD6_BCM1_0x216/FrWiperH ==
  FrWiperH : Inport
  Data Type Conversion : DataTypeConversion  OutDataTypeStr=uint8  RndMeth=Round
  CAN6_Fr_Wiper_H : Outport
  wires:
  Data Type Conversion/1 -> CAN6_Fr_Wiper_H/1
  FrWiperH/1 -> Data Type Conversion/1

== system halout/HAL_OUT/CAN6/FD6_BCM1_0x216/FrWiperL ==
  FrWiperL : Inport
  Data Type Conversion : DataTypeConversion  OutDataTypeStr=uint8  RndMeth=Round
  CAN6_Fr_Wiper_L : Outport
  wires:
  Data Type Conversion/1 -> CAN6_Fr_Wiper_L/1
  FrWiperL/1 -> Data Type Conversion/1

== system halout/HAL_OUT/CAN6/FD6_BCM1_0x216/HBeam ==
  HBeam : Inport
  Data Type Conversion : DataTypeConversion  OutDataTypeStr=uint8  RndMeth=Round
  CAN6_H_Beam : Outport
  wires:
  Data Type Conversion/1 -> CAN6_H_Beam/1
  HBeam/1 -> Data Type Conversion/1

== system halout/HAL_OUT/CAN6/FD6_BCM1_0x216/HazardSW ==
  HazardSW : Inport
  Data Type Conversion : DataTypeConversion  OutDataTypeStr=uint8  RndMeth=Round
  CAN6_HazardSW : Outport
  wires:
  Data Type Conversion/1 -> CAN6_HazardSW/1
  HazardSW/1 -> Data Type Conversion/1

== system halout/HAL_OUT/CAN6/FD6_BCM1_0x216/HoodSW ==
  HoodSW : Inport
  Data Type Conversion : DataTypeConversion  OutDataTypeStr=uint8  RndMeth=Round
  CAN6_HoodSW : Outport
  wires:
  Data Type Conversion/1 -> CAN6_HoodSW/1
  HoodSW/1 -> Data Type Conversion/1

== system halout/HAL_OUT/CAN6/FD6_BCM1_0x216/HornCtrl ==
  HornCtrl : Inport
  Data Type Conversion : DataTypeConversion  OutDataTypeStr=uint8  RndMeth=Round
  CAN6_HornCtrl : Outport
  wires:
  Data Type Conversion/1 -> CAN6_HornCtrl/1
  HornCtrl/1 -> Data Type Conversion/1

== system halout/HAL_OUT/CAN6/FD6_BCM1_0x216/LAPMWdwEnable ==
  LAPMWdwEnable : Inport
  Data Type Conversion : DataTypeConversion  OutDataTypeStr=uint8  RndMeth=Round
  CAN6_L_APM_WdwEnable : Outport
  wires:
  Data Type Conversion/1 -> CAN6_L_APM_WdwEnable/1
  LAPMWdwEnable/1 -> Data Type Conversion/1

== system halout/HAL_OUT/CAN6/FD6_BCM1_0x216/LBSD ==
  LBSD : Inport
  Data Type Conversion : DataTypeConversion  OutDataTypeStr=uint8  RndMeth=Round
  CAN6_LBSD : Outport
  wires:
  Data Type Conversion/1 -> CAN6_LBSD/1
  LBSD/1 -> Data Type Conversion/1

== system halout/HAL_OUT/CAN6/FD6_BCM1_0x216/LBeam ==
  LBeam : Inport
  Data Type Conversion : DataTypeConversion  OutDataTypeStr=uint8  RndMeth=Round
  CAN6_L_Beam : Outport
  wires:
  Data Type Conversion/1 -> CAN6_L_Beam/1
  LBeam/1 -> Data Type Conversion/1

== system halout/HAL_OUT/CAN6/FD6_BCM1_0x216/LDRL ==
  LDRL : Inport
  Data Type Conversion : DataTypeConversion  OutDataTypeStr=uint8  RndMeth=Round
  CAN6_LDRL : Outport
  wires:
  Data Type Conversion/1 -> CAN6_LDRL/1
  LDRL/1 -> Data Type Conversion/1

== system halout/HAL_OUT/CAN6/FD6_BCM1_0x216/LTurnLP ==
  LTurnLP : Inport
  Data Type Conversion : DataTypeConversion  OutDataTypeStr=uint8  RndMeth=Round
  CAN6_LTurnLP : Outport
  wires:
  Data Type Conversion/1 -> CAN6_LTurnLP/1
  LTurnLP/1 -> Data Type Conversion/1

== system halout/HAL_OUT/CAN6/FD6_BCM1_0x216/LockSetting ==
  LockSetting : Inport
  Data Type Conversion : DataTypeConversion  OutDataTypeStr=uint8  RndMeth=Round
  CAN6_LockSetting : Outport
  wires:
  Data Type Conversion/1 -> CAN6_LockSetting/1
  LockSetting/1 -> Data Type Conversion/1

== system halout/HAL_OUT/CAN6/FD6_BCM1_0x216/MirrorCtrl ==
  MirrorCtrl : Inport
  Data Type Conversion : DataTypeConversion  OutDataTypeStr=uint8  RndMeth=Round
  CAN6_MirrorCtrl : Outport
  wires:
  Data Type Conversion/1 -> CAN6_MirrorCtrl/1
  MirrorCtrl/1 -> Data Type Conversion/1

== system halout/HAL_OUT/CAN6/FD6_BCM1_0x216/MirrorDefog ==
  MirrorDefog : Inport
  Data Type Conversion : DataTypeConversion  OutDataTypeStr=uint8  RndMeth=Round
  CAN6_MirrorDefog : Outport
  wires:
  Data Type Conversion/1 -> CAN6_MirrorDefog/1
  MirrorDefog/1 -> Data Type Conversion/1

== system halout/HAL_OUT/CAN6/FD6_BCM1_0x216/PosLamp ==
  PosLamp : Inport
  Data Type Conversion : DataTypeConversion  OutDataTypeStr=uint8  RndMeth=Round
  CAN6_PosLamp : Outport
  wires:
  Data Type Conversion/1 -> CAN6_PosLamp/1
  PosLamp/1 -> Data Type Conversion/1

== system halout/HAL_OUT/CAN6/FD6_BCM1_0x216/PsDoorSW ==
  PsDoorSW : Inport
  Data Type Conversion : DataTypeConversion  OutDataTypeStr=uint8  RndMeth=Round
  CAN6_PsDoorSW : Outport
  wires:
  Data Type Conversion/1 -> CAN6_PsDoorSW/1
  PsDoorSW/1 -> Data Type Conversion/1

== system halout/HAL_OUT/CAN6/FD6_BCM1_0x216/RBSD ==
  RBSD : Inport
  Data Type Conversion : DataTypeConversion  OutDataTypeStr=uint8  RndMeth=Round
  CAN6_RBSD : Outport
  wires:
  Data Type Conversion/1 -> CAN6_RBSD/1
  RBSD/1 -> Data Type Conversion/1

== system halout/HAL_OUT/CAN6/FD6_BCM1_0x216/RDRL ==
  RDRL : Inport
  Data Type Conversion : DataTypeConversion  OutDataTypeStr=uint8  RndMeth=Round
  CAN6_RDRL : Outport
  wires:
  Data Type Conversion/1 -> CAN6_RDRL/1
  RDRL/1 -> Data Type Conversion/1

== system halout/HAL_OUT/CAN6/FD6_BCM1_0x216/RLDoorSW ==
  RLDoorSW : Inport
  Data Type Conversion : DataTypeConversion  OutDataTypeStr=uint8  RndMeth=Round
  CAN6_RLDoorSW : Outport
  wires:
  Data Type Conversion/1 -> CAN6_RLDoorSW/1
  RLDoorSW/1 -> Data Type Conversion/1

== system halout/HAL_OUT/CAN6/FD6_BCM1_0x216/RRDoorSW ==
  RRDoorSW : Inport
  Data Type Conversion : DataTypeConversion  OutDataTypeStr=uint8  RndMeth=Round
  CAN6_RRDoorSW : Outport
  wires:
  Data Type Conversion/1 -> CAN6_RRDoorSW/1
  RRDoorSW/1 -> Data Type Conversion/1

== system halout/HAL_OUT/CAN6/FD6_BCM1_0x216/RTurnLP ==
  RTurnLP : Inport
  Data Type Conversion : DataTypeConversion  OutDataTypeStr=uint8  RndMeth=Round
  CAN6_RTurnLP : Outport
  wires:
  Data Type Conversion/1 -> CAN6_RTurnLP/1
  RTurnLP/1 -> Data Type Conversion/1

== system halout/HAL_OUT/CAN6/FD6_BCM1_0x216/ReverseLamp ==
  ReverseLamp : Inport
  Data Type Conversion : DataTypeConversion  OutDataTypeStr=uint8  RndMeth=Round
  CAN6_ReverseLamp : Outport
  wires:
  Data Type Conversion/1 -> CAN6_ReverseLamp/1
  ReverseLamp/1 -> Data Type Conversion/1

== system halout/HAL_OUT/CAN6/FD6_BCM1_0x216/RoomLampH ==
  RoomLampH : Inport
  Data Type Conversion : DataTypeConversion  OutDataTypeStr=uint8  RndMeth=Round
  CAN6_RoomLampH : Outport
  wires:
  Data Type Conversion/1 -> CAN6_RoomLampH/1
  RoomLampH/1 -> Data Type Conversion/1

== system halout/HAL_OUT/CAN6/FD6_BCM1_0x216/RoomLampL ==
  RoomLampL : Inport
  Data Type Conversion : DataTypeConversion  OutDataTypeStr=uint8  RndMeth=Round
  CAN6_RoomLampL : Outport
  wires:
  Data Type Conversion/1 -> CAN6_RoomLampL/1
  RoomLampL/1 -> Data Type Conversion/1

== system halout/HAL_OUT/CAN6/FD6_BCM1_0x216/RrChargingDoorCtrl ==
  RrChargingDoorCtrl : Inport
  Data Type Conversion : DataTypeConversion  OutDataTypeStr=uint8  RndMeth=Round
  CAN6_Rr_ChargingDoorCtrl : Outport
  wires:
  Data Type Conversion/1 -> CAN6_Rr_ChargingDoorCtrl/1
  RrChargingDoorCtrl/1 -> Data Type Conversion/1

== system halout/HAL_OUT/CAN6/FD6_BCM1_0x216/RrDefog ==
  RrDefog : Inport
  Data Type Conversion : DataTypeConversion  OutDataTypeStr=uint8  RndMeth=Round
  CAN6_Rr_Defog : Outport
  wires:
  Data Type Conversion/1 -> CAN6_Rr_Defog/1
  RrDefog/1 -> Data Type Conversion/1

== system halout/HAL_OUT/CAN6/FD6_BCM1_0x216/RrFogLamp ==
  RrFogLamp : Inport
  Data Type Conversion : DataTypeConversion  OutDataTypeStr=uint8  RndMeth=Round
  CAN6_Rr_FogLamp : Outport
  wires:
  Data Type Conversion/1 -> CAN6_Rr_FogLamp/1
  RrFogLamp/1 -> Data Type Conversion/1

== system halout/HAL_OUT/CAN6/FD6_BCM1_0x216/RrWiper ==
  RrWiper : Inport
  Data Type Conversion : DataTypeConversion  OutDataTypeStr=uint8  RndMeth=Round
  CAN6_Rr_Wiper : Outport
  wires:
  Data Type Conversion/1 -> CAN6_Rr_Wiper/1
  RrWiper/1 -> Data Type Conversion/1

== system halout/HAL_OUT/CAN6/FD6_BCM1_0x216/TailgateHDSW ==
  TailgateHDSW : Inport
  Data Type Conversion : DataTypeConversion  OutDataTypeStr=uint8  RndMeth=Round
  CAN6_TailgateHDSW : Outport
  wires:
  Data Type Conversion/1 -> CAN6_TailgateHDSW/1
  TailgateHDSW/1 -> Data Type Conversion/1

== system halout/HAL_OUT/CAN6/FD6_BCM1_0x216/TailgateRemote ==
  TailgateRemote : Inport
  Data Type Conversion : DataTypeConversion  OutDataTypeStr=uint8  RndMeth=Round
  CAN6_TailgateRemote : Outport
  wires:
  Data Type Conversion/1 -> CAN6_TailgateRemote/1
  TailgateRemote/1 -> Data Type Conversion/1

== system halout/HAL_OUT/CAN6/FD6_BCM1_0x216/TailgateSW ==
  TailgateSW : Inport
  Data Type Conversion : DataTypeConversion  OutDataTypeStr=uint8  RndMeth=Round
  CAN6_Tailgate_SW : Outport
  wires:
  Data Type Conversion/1 -> CAN6_Tailgate_SW/1
  TailgateSW/1 -> Data Type Conversion/1

== system halout/HAL_OUT/CAN6/FD6_BCM1_0x216/TrunkRel ==
  TrunkRel : Inport
  Data Type Conversion : DataTypeConversion  OutDataTypeStr=uint8  RndMeth=Round
  CAN6_TrunkRel : Outport
  wires:
  Data Type Conversion/1 -> CAN6_TrunkRel/1
  TrunkRel/1 -> Data Type Conversion/1

== system halout/HAL_OUT/CAN6/FD6_BCM1_0x216/WasherCtrl ==
  WasherCtrl : Inport
  Data Type Conversion : DataTypeConversion  OutDataTypeStr=uint8  RndMeth=Round
  CAN6_WasherCtrl : Outport
  wires:
  Data Type Conversion/1 -> CAN6_WasherCtrl/1
  WasherCtrl/1 -> Data Type Conversion/1

== system halout/HAL_OUT/CAN6/FD6_BCM1_0x216/WiperFixMode ==
  WiperFixMode : Inport
  Data Type Conversion : DataTypeConversion  OutDataTypeStr=uint8  RndMeth=Round
  CAN6_WiperFixMode : Outport
  wires:
  Data Type Conversion/1 -> CAN6_WiperFixMode/1
  WiperFixMode/1 -> Data Type Conversion/1

== system halout/HAL_OUT/CAN6/FD6_VCU1_0x116/CCCrlSta ==
  CCCrlSta : Inport
  Data Type Conversion : DataTypeConversion  OutDataTypeStr=uint8  RndMeth=Round
  CAN6_CC_Crl_Sta : Outport
  wires:
  Data Type Conversion/1 -> CAN6_CC_Crl_Sta/1
  CCCrlSta/1 -> Data Type Conversion/1

== system halout/HAL_OUT/CAN6/FD6_VCU1_0x116/EngAGSCloseSta ==
  EngAGSCloseSta : Inport
  Data Type Conversion : DataTypeConversion  OutDataTypeStr=uint8  RndMeth=Round
  CAN6_Eng_AGSCloseSta : Outport
  wires:
  Data Type Conversion/1 -> CAN6_Eng_AGSCloseSta/1
  EngAGSCloseSta/1 -> Data Type Conversion/1

== system halout/HAL_OUT/CAN6/FD6_VCU1_0x116/EngActvDmpDisabSta ==
  EngActvDmpDisabSta : Inport
  Data Type Conversion : DataTypeConversion  OutDataTypeStr=uint8  RndMeth=Round
  CAN6_Eng_ActvDmpDisabSta : Outport
  wires:
  Data Type Conversion/1 -> CAN6_Eng_ActvDmpDisabSta/1
  EngActvDmpDisabSta/1 -> Data Type Conversion/1

== system halout/HAL_OUT/CAN6/FD6_VCU1_0x116/EngCoastDwSta ==
  EngCoastDwSta : Inport
  Data Type Conversion : DataTypeConversion  OutDataTypeStr=uint8  RndMeth=Round
  CAN6_Eng_CoastDwSta : Outport
  wires:
  Data Type Conversion/1 -> CAN6_Eng_CoastDwSta/1
  EngCoastDwSta/1 -> Data Type Conversion/1

== system halout/HAL_OUT/CAN6/FD6_VCU1_0x116/EngPwrLockSta ==
  EngPwrLockSta : Inport
  Data Type Conversion : DataTypeConversion  OutDataTypeStr=uint8  RndMeth=Round
  CAN6_Eng_PwrLockSta : Outport
  wires:
  Data Type Conversion/1 -> CAN6_Eng_PwrLockSta/1
  EngPwrLockSta/1 -> Data Type Conversion/1

== system halout/HAL_OUT/CAN6/FD6_VCU1_0x116/HVPwrSta ==
  HVPwrSta : Inport
  Data Type Conversion : DataTypeConversion  OutDataTypeStr=uint8  RndMeth=Round
  CAN6_HVPwrSta : Outport
  wires:
  Data Type Conversion/1 -> CAN6_HVPwrSta/1
  HVPwrSta/1 -> Data Type Conversion/1

== system halout/HAL_OUT/CAN6/FD6_VCU1_0x116/LVPwrSta ==
  LVPwrSta : Inport
  Data Type Conversion : DataTypeConversion  OutDataTypeStr=uint8  RndMeth=Round
  CAN6_LVPwrSta : Outport
  wires:
  Data Type Conversion/1 -> CAN6_LVPwrSta/1
  LVPwrSta/1 -> Data Type Conversion/1

== system halout/HAL_OUT/CAN6/FD6_VCU1_0x116/MSACrlSta ==
  MSACrlSta : Inport
  Data Type Conversion : DataTypeConversion  OutDataTypeStr=uint8  RndMeth=Round
  CAN6_MSA_Crl_Sta : Outport
  wires:
  Data Type Conversion/1 -> CAN6_MSA_Crl_Sta/1
  MSACrlSta/1 -> Data Type Conversion/1

== system halout/HAL_OUT/CAN6/FD6_VCU1_0x116/PButtonSta ==
  PButtonSta : Inport
  Data Type Conversion : DataTypeConversion  OutDataTypeStr=uint8  RndMeth=Round
  CAN6_P_Button_Sta : Outport
  wires:
  Data Type Conversion/1 -> CAN6_P_Button_Sta/1
  PButtonSta/1 -> Data Type Conversion/1

== system halout/HAL_OUT/CAN6/FD6_VCU1_0x116/PrkReq ==
  PrkReq : Inport
  Data Type Conversion : DataTypeConversion  OutDataTypeStr=uint8  RndMeth=Round
  CAN6_PrkReq : Outport
  wires:
  Data Type Conversion/1 -> CAN6_PrkReq/1
  PrkReq/1 -> Data Type Conversion/1

== system halout/HAL_OUT/CAN6/FD6_VCU1_0x116/PrkReqValid ==
  PrkReqValid : Inport
  Data Type Conversion : DataTypeConversion  OutDataTypeStr=uint8  RndMeth=Round
  CAN6_PrkReqValid : Outport
  wires:
  Data Type Conversion/1 -> CAN6_PrkReqValid/1
  PrkReqValid/1 -> Data Type Conversion/1

== system halout/HAL_OUT/CAN6/FD6_VCU1_0x116/PwrSta ==
  PwrSta : Inport
  Data Type Conversion : DataTypeConversion  OutDataTypeStr=uint8  RndMeth=Round
  CAN6_PwrSta : Outport
  wires:
  Data Type Conversion/1 -> CAN6_PwrSta/1
  PwrSta/1 -> Data Type Conversion/1

== system halout/HAL_OUT/CAN6/FD6_VCU1_0x116/ShiftGearPosn ==
  ShiftGearPosn : Inport
  Data Type Conversion : DataTypeConversion  OutDataTypeStr=uint8  RndMeth=Round
  CAN6_ShiftGearPosn : Outport
  wires:
  Data Type Conversion/1 -> CAN6_ShiftGearPosn/1
  ShiftGearPosn/1 -> Data Type Conversion/1

== system halout/HAL_OUT/CAN6/FD6_VCU1_0x116/VCUOPDHold ==
  VCUOPDHold : Inport
  Data Type Conversion : DataTypeConversion  OutDataTypeStr=uint8  RndMeth=Round
  CAN6_VCU_OPDHold : Outport
  wires:
  Data Type Conversion/1 -> CAN6_VCU_OPDHold/1
  VCUOPDHold/1 -> Data Type Conversion/1

== system halout/HAL_OUT/CAN6/FD6_VCU1_0x116/VehMalfunLevel ==
  VehMalfunLevel : Inport
  Data Type Conversion : DataTypeConversion  OutDataTypeStr=uint8  RndMeth=Round
  CAN6_VehMalfunLevel : Outport
  wires:
  Data Type Conversion/1 -> CAN6_VehMalfunLevel/1
  VehMalfunLevel/1 -> Data Type Conversion/1

== system halout/HAL_OUT/CAN6/FD6_VCU1_0x116/XWDMode ==
  XWDMode : Inport
  Data Type Conversion : DataTypeConversion  OutDataTypeStr=uint8  RndMeth=Round
  CAN6_XWDMode : Outport
  wires:
  Data Type Conversion/1 -> CAN6_XWDMode/1
  XWDMode/1 -> Data Type Conversion/1

== system halout/HAL_OUT/CAN6/FD6_VCU2_0x154/ACCCtrlAvail ==
  ACCCtrlAvail : Inport
  Data Type Conversion : DataTypeConversion  OutDataTypeStr=uint8  RndMeth=Round
  CAN6_ACC_CtrlAvail : Outport
  wires:
  Data Type Conversion/1 -> CAN6_ACC_CtrlAvail/1
  ACCCtrlAvail/1 -> Data Type Conversion/1

== system halout/HAL_OUT/CAN6/FD6_VCU2_0x154/AccPedalOverride ==
  AccPedalOverride : Inport
  Data Type Conversion : DataTypeConversion  OutDataTypeStr=uint8  RndMeth=Round
  CAN6_AccPedal_Override : Outport
  wires:
  Data Type Conversion/1 -> CAN6_AccPedal_Override/1
  AccPedalOverride/1 -> Data Type Conversion/1

== system halout/HAL_OUT/CAN6/FD6_VCU2_0x154/ActAPSPosn ==
  ActAPSPosn : Inport
  Data Type Conversion : DataTypeConversion  OutDataTypeStr=uint8  RndMeth=Round
  convert_out : FVT_lib/hal/convert_out  gain=0.394  offset=0
  CAN6_ActAPSPosn : Outport
  wires:
  Data Type Conversion/1 -> CAN6_ActAPSPosn/1
  convert_out/1 -> Data Type Conversion/1
  ActAPSPosn/1 -> convert_out/1

== system halout/HAL_OUT/CAN6/FD6_VCU2_0x154/Byte_0 ==
  CS_VCU2_CAN6 : Inport
  BitwiseOR : simulink/Logic and Bit Operations/Bitwise Operator  logicop=OR  UseBitMask=off  BitMask=bin2dec('11011001')  BitMaskRealWorld=Stored Integer
  SignalPack : FVT_lib/hal/SignalPack  RightShiftCnt=0  BitMask=2^8-1  LeftShiftCnt=0
  UnitConverter : DataTypeConversion  OutDataTypeStr=uint8  RndMeth=Round
  UnitConverter1 : DataTypeConversion  OutDataTypeStr=uint8  RndMeth=Round
  Byte_0 : Outport
  wires:
  BitwiseOR/1 -> Byte_0/1
  UnitConverter/1 -> BitwiseOR/1
  SignalPack/1 -> UnitConverter/1
  UnitConverter1/1 -> SignalPack/1
  CS_VCU2_CAN6/1 -> UnitConverter1/1

== system halout/HAL_OUT/CAN6/FD6_VCU2_0x154/Byte_1 ==
  RC_VCU2_CAN6 : Inport
  BitwiseOR : simulink/Logic and Bit Operations/Bitwise Operator  logicop=OR  UseBitMask=off  BitMask=bin2dec('11011001')  BitMaskRealWorld=Stored Integer
  SignalPack : FVT_lib/hal/SignalPack  RightShiftCnt=0  BitMask=2^4-1  LeftShiftCnt=0
  UnitConverter : DataTypeConversion  OutDataTypeStr=uint8  RndMeth=Round
  UnitConverter1 : DataTypeConversion  OutDataTypeStr=uint8  RndMeth=Round
  Byte_1 : Outport
  wires:
  BitwiseOR/1 -> Byte_1/1
  UnitConverter/1 -> BitwiseOR/1
  SignalPack/1 -> UnitConverter/1
  UnitConverter1/1 -> SignalPack/1
  RC_VCU2_CAN6/1 -> UnitConverter1/1

== system halout/HAL_OUT/CAN6/FD6_VCU2_0x154/Byte_10 ==
  VehActPwr : Inport
  BitwiseOR : simulink/Logic and Bit Operations/Bitwise Operator  logicop=OR  UseBitMask=off  BitMask=bin2dec('11011001')  BitMaskRealWorld=Stored Integer
  SignalPack : FVT_lib/hal/SignalPack  RightShiftCnt=16  BitMask=2^8-1  LeftShiftCnt=0
  UnitConverter : DataTypeConversion  OutDataTypeStr=uint8  RndMeth=Round
  UnitConverter1 : DataTypeConversion  OutDataTypeStr=uint32  RndMeth=Round
  convert_out : FVT_lib/hal/convert_out  gain=1  offset=-600000
  Byte_10 : Outport
  wires:
  BitwiseOR/1 -> Byte_10/1
  UnitConverter/1 -> BitwiseOR/1
  SignalPack/1 -> UnitConverter/1
  UnitConverter1/1 -> SignalPack/1
  convert_out/1 -> UnitConverter1/1
  VehActPwr/1 -> convert_out/1
